simulink model "lowpassRCFilter_R24b_panels"  (R2024b)
settings: Solver=VariableStepAuto  StartTime=0.0  StopTime=inf  RelTol=1e-3  AbsTol=1e-3
libraries: nesl_utility x5, fl_lib x4, ee_lib x1
settings Model: PacingRate=0.100000  Creator=clapierr  LastModifiedBy=clapierr
settings SolverCC: AutoScaleAbsTol=off  AlgebraicLoopSolver=TrustRegion  MaxZcPerStep=1
settings DebuggingCC: UnconnectedInputMsg=warning  UnconnectedOutputMsg=warning  UnconnectedLineMsg=warning  SymbolicDimsDataTypeCodeGenerationDiagnostic=none
settings ModelReferenceCC: EnableRefExpFcnMdlSchedulingChecks=on
settings SFSimCC: CustomCodeUndefinedFunction=UseInterfaceOnly
settings RTWCC: GPUComputeCapability=3.5  DLArmComputeVersion=19.05
settings SimscapeCC: SimscapeLogType=local  SimscapeLogLimitData=off  SimscapeLogDataHistory=10000

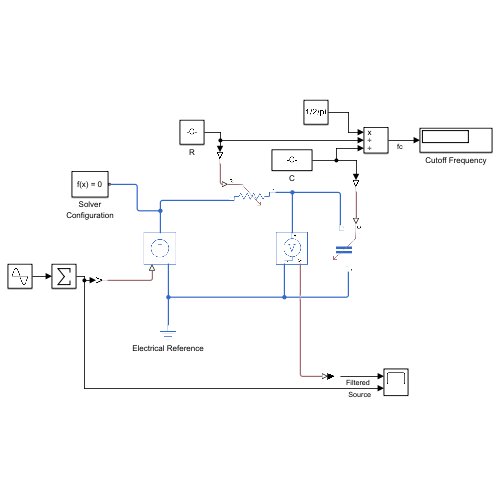
[thumbnail: Simulink's stored preview of the top-level diagram]
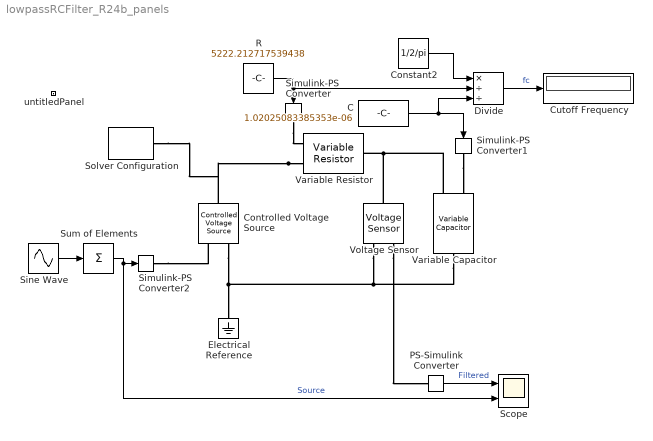
== system lowpassRCFilter_R24b_panels ==
  C : Constant  Value=1.02025083385353e-06
  Constant2 : Constant  Value=1/2/pi
  Controlled Voltage Source : fl_lib/Electrical/Electrical Sources/Controlled Voltage Source
  Cutoff Frequency : Display
  Divide : Product  Inputs=*//
  Electrical Reference : fl_lib/Electrical/Electrical Elements/Electrical Reference
  PS-Simulink Converter : nesl_utility/PS-Simulink Converter  PhysicalDomain=network_engine_domain  SubClassName=ps_output  LeftPortType=input  RightPortType=output  PseudoPeriodic=off  Frequencies=[]  VectorFormat=inherit  Unit=inherit  AffineConversion=off
  R : Constant  Value=5222.212717539438
  Scope : Scope  NumInputPorts=2
  Simulink-PS Converter : nesl_utility/Simulink-PS Converter  PhysicalDomain=network_engine_domain  SubClassName=ps_input  LeftPortType=input  RightPortType=output  PseudoPeriodic=off  Frequencies=[]  NoiseDistribution=none  NoiseParameters=[]  Unit=Ohm  AffineConversion=off  FilteringAndDerivatives=provide  SimscapeFilterOrder=1  InputFilterTimeConstant=0.001  UdotUserProvided=0
  Simulink-PS Converter1 : nesl_utility/Simulink-PS Converter  PhysicalDomain=network_engine_domain  SubClassName=ps_input  LeftPortType=input  RightPortType=output  PseudoPeriodic=off  Frequencies=[]  NoiseDistribution=none  NoiseParameters=[]  Unit=F  AffineConversion=off  FilteringAndDerivatives=provide  SimscapeFilterOrder=1  InputFilterTimeConstant=0.001  UdotUserProvided=0
  Simulink-PS Converter2 : nesl_utility/Simulink-PS Converter  PhysicalDomain=network_engine_domain  SubClassName=ps_input  LeftPortType=input  RightPortType=output  PseudoPeriodic=off  Frequencies=[]  NoiseDistribution=none  NoiseParameters=[]  Unit=1  AffineConversion=off  FilteringAndDerivatives=provide  SimscapeFilterOrder=1  InputFilterTimeConstant=0.001  UdotUserProvided=0
  Sine Wave : Sin  Amplitude=[1 0.1]  Frequency=2*pi*[10 60]  SampleTime=0
  Solver Configuration : nesl_utility/Solver Configuration  PhysicalDomain=network_engine_domain  SubClassName=solver  LeftPortType=input  RightPortType=generic  Tones=[]  Harmonics=[]  SimulateNoise=off  Profile=off  UseLocalSampling=off  EnableSwitchedLinearOptims=on  FrequencyDomain=off  UseCCode=off  RelTol=0.001  AbsTol=1e-06  MinStep=1e-09  ToWorkspace=off  RevertToSquareIcSolve=off  NumHomotopyIterations=100  PhasorMode=off  PhasorModeNumHarmonics=1  ConsistencySolver=NEWTON_XTOL_AFTER_FTOL  IndexReductionMethod=DerivativeReplacement  DoDC=off  ResidualTolerance=1e-09  ConsistencyTolSource=GLOBAL  ConsistencyAbsTol=0.001  ConsistencyRelTol=0.001  ConsistencyTolFactor=0.001  UseLocalSolver=off  LocalSolverChoice=NE_BACKWARD_EULER_ADVANCER  ResolveIndetEquations=on  FunctionEvalNumThread=1  LocalSolverSampleTime=1e-5  DoFixedCost=off  MaxNonlinIter=3  MaxModeIter=2  ComputeImpulses=off  ImpulseIterations=2  LinearAlgebra=auto  LinearAlgebraNumThread=0  EquationFormulation=NE_TIME_EF  DelaysMemoryBudget=1024  AutomaticFiltering=on  FilteringTimeConstant=0.001  PartitionStorageMethod=AS_NEEDED  PartitionMemoryBudget=1024  PartitionMethod=ROBUST  MultibodyUseLocalSolver=off  MultibodyLocalSolverChoice=ODE1  MultibodyLocalSolverSampleTime=0.001
  Sum of Elements : Sum  Inputs=+
  Variable Capacitor : ee_lib/Passive/Variable Capacitor  prm=2  Cmin=1e-12 F  r=1e-6 Ohm  v0=0 V  q0=0 C
      settings: InternalSimscapePortConfiguration="{\"Bottom\":[],\"Left\":[{\"id\":\"C\",\"label\":\"C\",\"type\":\"input\"},{\"id\":\"p\",\"label\":\"+\",\"type\":\"foundation.electrical.electrical\"}],\"Right\":[{\"id\":\"n\",\"label\":\"-\",\"type\":\"foundation.electrical.electrical\"}],\"Top\":[]}"
  Variable Resistor : fl_lib/Electrical/Electrical Elements/Variable Resistor  Rmin=0 Ohm  thermalEnable=false  thermal_mass=1 J/K  i_specify=off  i_priority=None  i=0 A  i_nominal_specify=off  i_nominal_value=1  i_nominal_unit=A  v_specify=off  v_priority=None  v=0 V  v_nominal_specify=off  v_nominal_value=1  v_nominal_unit=V  T_specify=off  T_priority=None  T=300 K  T_nominal_specify=off  T_nominal_value=1  T_nominal_unit=K
  Voltage Sensor : fl_lib/Electrical/Electrical Sensors/Voltage Sensor
  untitledPanel : Subsystem  Tag=HiddenForWebPanel  IsWebBlockPanel=on
  wires:
  Sum of Elements/1 -> Scope/2, Simulink-PS Converter2/1  "Source"
  PS-Simulink Converter/1 -> Scope/1  "Filtered"
  R/1 -> Simulink-PS Converter/1, Divide/2
  C/1 -> Simulink-PS Converter1/1, Divide/3
  Sine Wave/1 -> Sum of Elements/1
  Constant2/1 -> Divide/1
  Divide/1 -> Cutoff Frequency/1  "fc"
  connections:
  Voltage Sensor/LConn1 -- Variable Resistor/RConn1 -- Variable Capacitor/LConn2
  Voltage Sensor/RConn2 -- Controlled Voltage Source/RConn2 -- Electrical Reference/LConn1 -- Variable Capacitor/RConn1
  Variable Resistor/LConn2 -- Solver Configuration/RConn1 -- Controlled Voltage Source/LConn1
  Voltage Sensor/RConn1 -- PS-Simulink Converter/LConn1
  Simulink-PS Converter/RConn1 -- Variable Resistor/LConn1
  Simulink-PS Converter1/RConn1 -- Variable Capacitor/LConn1
  Simulink-PS Converter2/RConn1 -- Controlled Voltage Source/RConn1

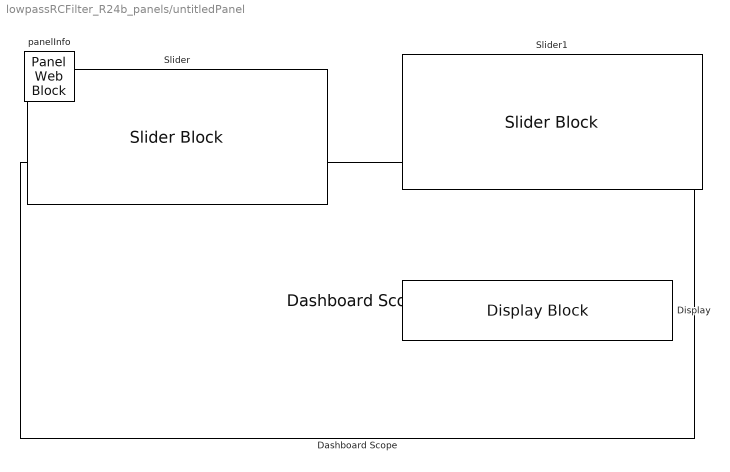
== system lowpassRCFilter_R24b_panels/untitledPanel ==
  Dashboard Scope : DashboardScope  Tag=HiddenForWebPanel  PanelInfo="{\"height\":386,\"left\":11,\"panelId\":\"panelId-89ad8147-c2ec-492f-99dc-ed40cfdb93ef\",\"top\":15,\"type\":\"panelChild\",\"version\":\"2019b\",\"width\":682,\"zIndex\":1500014}"  TimeSpan=1  Ymin=-2  Ymax=2  ScaleAtStop=off  UpdateMode=Scroll
  Display : DisplayBlock  Tag=HiddenForWebPanel  PanelInfo="{\"height\":52,\"left\":24,\"panelId\":\"panelId-89ad8147-c2ec-492f-99dc-ed40cfdb93ef\",\"top\":602,\"type\":\"panelChild\",\"version\":\"2019b\",\"width\":147,\"zIndex\":1500010}"  Format=Custom  Transparency=1  FormatString=%.0f
  Slider : SliderBlock  Tag=HiddenForWebPanel  PanelInfo="{\"height\":68,\"left\":15,\"panelId\":\"panelId-89ad8147-c2ec-492f-99dc-ed40cfdb93ef\",\"top\":425,\"type\":\"panelChild\",\"version\":\"2019b\",\"width\":677,\"zIndex\":1500012}"  ScaleMin=100  ScaleMax=10000
  Slider1 : SliderBlock  Tag=HiddenForWebPanel  PanelInfo="{\"height\":63,\"left\":18,\"panelId\":\"panelId-89ad8147-c2ec-492f-99dc-ed40cfdb93ef\",\"top\":514,\"type\":\"panelChild\",\"version\":\"2019b\",\"width\":671,\"zIndex\":1500006}"  ScaleMin=1e-8  ScaleMax=1e-4  ScaleType=Log
  panelInfo : PanelWebBlock  Tag=HiddenForWebPanel  PanelInfo="{\"compacted\":false,\"height\":677,\"isActiveTab\":true,\"left\":1055,\"name\":\"Panel\",\"panelId\":\"panelId-89ad8147-c2ec-492f-99dc-ed40cfdb93ef\",\"popoutData\":{\"height\":0,\"left\":0,\"maximized\":false,\"top\":0,\"width\":0},\"popoutMode\":\"component\",\"tabIndex\":0,\"tabbedSetId\":\"tabbedSet8050616155\",\"top\":48,\"type\":\"panel\",\"version\":\"2019b\",\"visible\":true,\"width\":710,\"zIndex\":1500002}"  PanelSnapshot=<binary blob, 12352 chars, not shown>
